simulink model "test12_sudu_pmx_2020a_1"  (R2020a)
settings: Solver=VariableStepAuto  StartTime=0.0  StopTime=100  RelTol=1e-5  AbsTol=1e-5
undefined symbols (not defined in the file or in its folder): Earth, js_decode, js_encode, sigbuilder_block, WGS84
libraries: simulink x14, simulink_extras x7, aerolibfltsims x2, instrumentlib x2, shared6dof x1, aerolibasang x1, aerolibtransform2 x1, aerolibanimutils x1, dspnetwork x1
settings Model: Creator=mx  LastModifiedBy=Platform

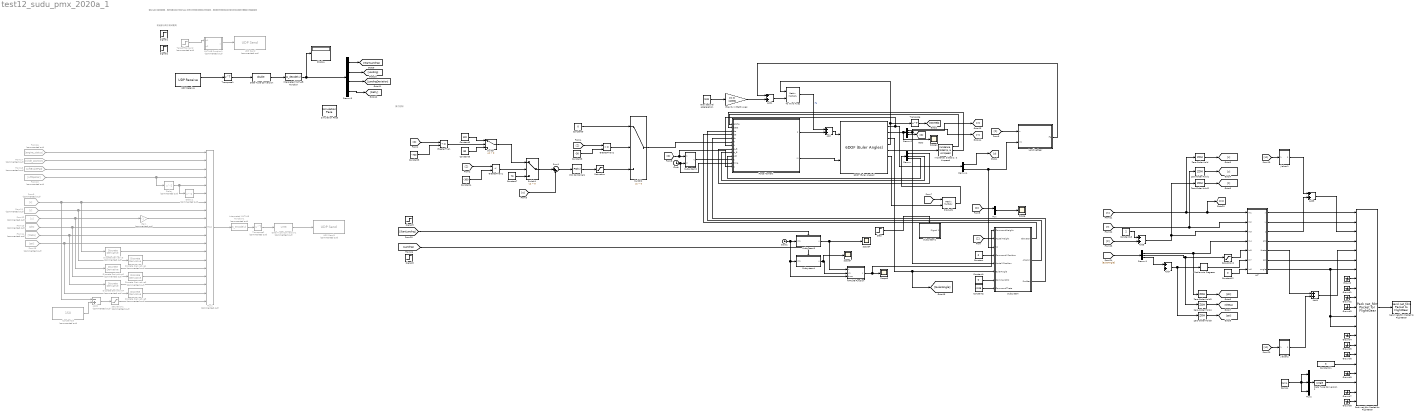
== system test12_sudu_pmx_2020a_1 ==
  note: 推力控制
  note: 通过UDP接收数据，暂时通过自己创造Json的形式来测试是否正常接收，联调的时候将此区域内的发送部分删除只保留接收
  note: 发送部分用于测试使用
  6DOF (Euler Angles) : shared6dof/6DOF (Euler Angles)  units=Metric (MKS)  mtype=Fixed  rep=Euler Angles  xme_0=[0 0 -600]  Vm_0=[80*cosd(-0) 0 80*sind(-0)]  eul_0=[0 -0*pi/180 0]  pm_0=[0 0 0]  mass_0=11000  mass_e=0.5  mass_f=2.0  inertia=[1000,0,0;0,2000,0;0,0,1000]  inertia_e=eye(3)  inertia_f=2*eye(3)  k_quat=1.0  vre_flag=on  abi_flag=off  aMode=0  xme_statename=''  Vm_statename=''  eul_statename=''  quat_statename=''  pm_statename=''  mass_statename=''
      settings: SourceProductBaseCode=AE,PW,MT,UV,VE,VP
  Add{,1,3..5,7} (6 alike) : Sum
  Add2 : Sum  Commented=on  Inputs=-+
  Clock : Clock
  Clock1 : Clock
  Constant{,1,9,12} (4 alike) : Constant  Value=0
  Constant10 : Constant  Commented=on  Value=150
  Constant11 : Constant  Value=3  OutDataTypeStr=uint32
  Constant13 : Constant  Value=2
  Constant2 : Constant  Value=-0.06
  Constant3 : Constant  Value=-700
  Constant4 : Constant  Value=-300
  Constant5 : Constant  Value=80
  Constant6 : Constant  Value=120
  Constant7 : Constant  Value=70
  Constant8 : Constant  Value=-30
  Data Type Conversion : DataTypeConversion  OutDataTypeStr=double
  Data Type Conversion1 : DataTypeConversion  Commented=on  OutDataTypeStr=uint8
  Data Type Conversion2 : DataTypeConversion  OutDataTypeStr=single
  Delay : Delay  Commented=on  InitialCondition=0  SampleTime=1
  Delay1 : Delay  Commented=on  InitialCondition=0  SampleTime=1
  Demux{,1..2,4} (4 alike) : Demux  Outputs=3
  Demux3 : Demux
  Discrete Derivative{,1..5} (6 alike) : simulink/Discrete/Discrete Derivative  Commented=on  gainval=1.0  ICPrevScaledInput=0.0  OutMin=[]  OutMax=[]  OutDataType=fixdt(1, 16)  OutScaling=2^-10  DoSatur=off
  Display : Display
  Force Moment : MATLAB Function  TreatAsAtomicUnit=on
  From10 : From  Commented=on  GotoTag=LiftSpoiler
  From11 : From  Commented=on  GotoTag=y
  From12 : From  Commented=on  GotoTag=z
  From13 : From  Commented=on  GotoTag=phi
  From14 : From  Commented=on  GotoTag=theta
  From15 : From  Commented=on  GotoTag=psi
  From16 : From  Commented=on  GotoTag=engine_status
  From17 : From  Commented=on  GotoTag=slide_position
  From18 : From  Commented=on  GotoTag=LiftBrakePad
  From9 : From  Commented=on  GotoTag=x
  Gain : Gain  Commented=on  Gain=-1
  Gravitational acceleration : Constant  Value=9.81
  Gravity in Earth Axes : Gain  Gain=[0; 0; 11000]  SaturateOnIntegerOverflow=on  OutDataTypeStr=Inherit: Same as input  ParamDataTypeStr=Inherit: Same as input
  GreaterThan : RelationalOperator  Operator=<=  OutDataTypeStr=boolean  RndMeth=Simplest
  GreaterThan1 : RelationalOperator  Operator=<  OutDataTypeStr=boolean  RndMeth=Simplest
  GreaterThan2 : RelationalOperator  OutDataTypeStr=boolean  RndMeth=Simplest
  Ground{,1..9} (10 alike) : Ground
  "Incidence, Sideslip, & Airspeed" : aerolibasang/Incidence, Sideslip, & Airspeed
  Interpreted MATLAB Function : MATLABFcn  MATLABFcn=js_decode(u)
  Interpreted MATLAB Function1 : MATLABFcn  Commented=on  MATLABFcn=js_encode(u)
  LLT : Subsystem
  LandingGear : MATLAB Function  TreatAsAtomicUnit=on
  MATLAB Function : MATLAB Function  TreatAsAtomicUnit=on
  MATLAB Function1 : MATLAB Function  Commented=on  TreatAsAtomicUnit=on
  Mux : Mux  Inputs=2
  Mux1 : Mux  Commented=on  Inputs=19
  Mux2 : Mux  Inputs=3
  PID Controller1 : simulink/Continuous/PID Controller  Controller=PID  Form=Parallel  TimeDomain=Continuous-time  UseExternalTs=off  SampleTime=-1  IntegratorMethod=Forward Euler  FilterMethod=Forward Euler  ControllerParametersSource=internal  P=100000  I=5000  D=10  UseFilter=on  N=10/10  TunerSelectOption=Transfer Function Based (PID Tuner App)  InitialConditionSource=internal  InitialConditionForIntegrator=0  InitialConditionForFilter=0  DifferentiatorICPrevScaledInput=0  ExternalReset=none  TrackingMode=off  Kt=1  LimitOutput=off  UpperSaturationLimit=inf  LowerSaturationLimit=-inf  LinearizeAsGain=on  AntiWindupMode=none  Kb=1  POutMin=[]  POutMax=[]  IOutMin=[]  IOutMax=[]  DOutMin=[]  DOutMax=[]  NOutMin=[]  NOutMax=[]  SumOutMin=[]  SumOutMax=[]  SaturationOutMin=[]  SaturationOutMax=[]  PParamMin=[]  PParamMax=[]  IParamMin=[]  IParamMax=[]  DParamMin=[]  DParamMax=[]  NParamMin=[]  NParamMax=[]  KbParamMin=[]  KbParamMax=[]  KtParamMin=[]  KtParamMax=[]  KbOutMin=[]  KbOutMax=[]  KtOutMin=[]  KtOutMax=[]  IntegratorOutMin=[]  IntegratorOutMax=[]  FilterOutMin=[]  FilterOutMax=[]  SumI1OutMin=[]  SumI1OutMax=[]  SumI2OutMin=[]  SumI2OutMax=[]  SumI3OutMin=[]  SumI3OutMax=[]  SumI4OutMin=[]  SumI4OutMax=[]  SumDOutMin=[]  SumDOutMax=[]  DifferentiatorOutMin=[]  DifferentiatorOutMax=[]  FilterDiffOutCoefMin=[]  FilterDiffOutCoefMax=[]  ReciprocalOutMin=[]  ReciprocalOutMax=[]  SumDenOutMin=[]  SumDenOutMax=[]  SumNumOutMin=[]  SumNumOutMax=[]  DivideOutMin=[]  DivideOutMax=[]  UdiffTsProdOutMin=[]  UdiffTsProdOutMax=[]  NTsProdOutMin=[]  NTsProdOutMax=[]  UintegralTsProdOutMin=[]  UintegralTsProdOutMax=[]  UngainTsProdOutMin=[]  UngainTsProdOutMax=[]  IntegratorContinuousStateAttributes=''  IntegratorStateMustResolveToSignalObject=off  IntegratorRTWStateStorageClass=Auto  FilterContinuousStateAttributes=''  FilterStateMustResolveToSignalObject=off  FilterRTWStateStorageClass=Auto  ParallelPVariant=InternalParameters  IdealPVariant=Disabled  IVariant=InternalParameters  DVariant=InternalParameters  IntegratorVariant=Continuous  SatVariant=Disabled  AWVariant=Passthrough  PCopyVariant=Disabled  TRVariant=Disabled  FdbkBlocksVariant=Forward  IdealPFdbkVariant=Disabled  SatFdbkVariant=Disabled  DerivativeFilterVariant=ContFilter  NVariant=InternalParameters  NCopyVariant=Disabled  FilterICVariant=InternalICsFilter  IntegratorICVariant=InternalICs  ExternalResetVariant=Disabled  TRSumVariant=Passthrough  SumFdbkVariant=Disabled  SumVariant=Sum_PID  TsampFilterVariant=InternalTs  TsampNgainVariant=Passthrough  TsampIntegralVariant=Passthrough
  Pack net_fdm Packet for FlightGear : aerolibfltsims/Pack net_fdm Packet for FlightGear  FlightGearVersion=v2.12  ShowPositionAttitudeInputs=on  ShowVelocityAccelerationInputs=off  ShowControlSurfacePositionInputs=on  ShowEngineFuelInputs=off  ShowLandingGearInputs=on  ShowEnvironmentInputs=off  SampleTime=1/30  packetVersion=24
      settings: SourceProductBaseCode=AE
  Product1 : Product  Multiplication=Matrix(*)
  Radians to Degrees : simulink_extras/Transformations/Radians to Degrees
  Ramp4 : simulink/Sources/Ramp  slope=-0.2  start=20  InitialOutput=1
  Saturation : Saturate  UpperLimit=40000  LowerLimit=0
  Saturation1 : Saturate  Commented=on  UpperLimit=150  LowerLimit=0
  Saturation2 : Saturate  UpperLimit=20
  Scope{,1,3..4,7} (5 alike) : Scope
  Send net_fdm Packet to FlightGear : aerolibfltsims/Send net_fdm Packet to FlightGear  DestinationIpAddress=127.0.0.1  DestinationPort=5502  LocalIpPort=-1  varLen=off  SampleTime=1/30
      settings: SourceProductBaseCode=AE
  Signal1 : Step  Time=2  SampleTime=0
  Signal2 : Step  Time=45  SampleTime=0
  Signal5 : Step  Time=2  SampleTime=0
  Signal8 : Step  Time=45  SampleTime=0
  Simulation Pace : aerolibanimutils/Simulation Pace  SimulationPace=1  SleepMode=Auto  OutputPaceError=off  SampleTime=1
  Step : Step  After=2  SampleTime=0
  Subsystem : Subsystem
  Subsystem1 : Subsystem
  Subsystem2 : Subsystem
  Subsystem3 : Subsystem
  Subsystem4 : Subsystem
  Sum1 : Sum  Inputs=|+-
  Switch : Switch  Criteria=u2 > Threshold
  Switch1 : Switch  Criteria=u2 > Threshold
  Switch2 : Switch  Criteria=u2 > Threshold
  TakeOffComand : Step  Commented=on  Time=6  SampleTime=1
  To Wind Axes : Product  Multiplication=Matrix(*)  InputSameDT=on  SaturateOnIntegerOverflow=on  OutDataTypeStr=Inherit: Same as first input
  Transpose : Math  Operator=transpose  SaturateOnIntegerOverflow=on
  Transpose1 : Math  Operator=transpose  SignedPower=on  SaturateOnIntegerOverflow=on
  Transpose2 : Math  Commented=on  Operator=transpose  SaturateOnIntegerOverflow=on
  UDP Receive : dspnetwork/UDP Receive  localURL='0.0.0.0'  localPort=51001  remoteURL='0.0.0.0'  remotePort=-1  recvBufferSize=8192  dims=992  signalDatatype=uint8  isComplex=off  isVarSize=off  showBlockingTime=off  blockingTime=0  sampletime=1  blockPlatform=[]
  UDP Send : instrumentlib/UDP Send  Commented=on  Host=localhost  Port=51001  LocalPort=-1  EnablePortSharing=off  ByteOrder=BigEndian  OutputDatagramPacketSize=996  EnableBlockingMode=on  LocalAddress=0.0.0.0
  UDP Send1 : instrumentlib/UDP Send  Commented=on  Host=localhost  Port=51003  LocalPort=-1  EnablePortSharing=off  ByteOrder=BigEndian  OutputDatagramPacketSize=1147  EnableBlockingMode=on  LocalAddress=0.0.0.0
  Zero-Order Hold{,1..5} (6 alike) : ZeroOrderHold  SampleTime=-1
  jiaban1 : Subsystem
  jiaban2 : Subsystem
  wires:
  Force Moment/2(M) -> 6DOF (Euler Angles)/2
  6DOF (Euler Angles)/5 -> "Incidence, Sideslip, & Airspeed"/1
  Gravitational acceleration/1 -> Gravity in Earth Axes/1
  To Wind Axes/1 -> Add/1  "Fg"
  Force Moment/1(F) -> Add/2
  Add/1 -> 6DOF (Euler Angles)/1
  "Incidence, Sideslip, & Airspeed"/1 -> Force Moment/1(alpha)
  "Incidence, Sideslip, & Airspeed"/2 -> Force Moment/2(beta)
  6DOF (Euler Angles)/1 -> Demux4/1, Force Moment/7(V)
  Demux/2 -> Force Moment/9(q_B)
  6DOF (Euler Angles)/2 -> Scope1/1, Demux2/1
  6DOF (Euler Angles)/3 -> [EulerAngle], Subsystem/6(EulerAngle)
  Demux4/3 -> LandingGear/2(Vz), Subsystem/3(Vz)
  Mux/1 -> Scope/1
  Constant/1 -> Subsystem/4(CommandYPosition)
  Demux2/2 -> [Y], Subsystem/5(AcutalYPosition)
  Constant1/1 -> Subsystem/7(CommandPsi)
  Constant2/1 -> Subsystem/8(CommandTheta)
  Demux2/3 -> [Z]
  [Z] -> Subsystem/2(AcutalHeight)
  [Z] -> GreaterThan/1
  Constant3/1 -> GreaterThan/2
  Constant4/1 -> GreaterThan1/2
  [Z] -> GreaterThan1/1
  GreaterThan/1 -> Switch/2
  Constant5/1 -> Switch/3
  Constant6/1 -> Switch/1
  GreaterThan1/1 -> Switch1/2
  Constant7/1 -> Switch1/3
  Switch/1 -> Switch1/1
  Switch1/1 -> Sum1/1
  Sum1/1 -> PID Controller1/1
  Demux4/1 -> [u]
  [u] -> Sum1/2
  PID Controller1/1 -> Saturation/1
  Saturation/1 -> Switch2/3
  Constant8/1 -> GreaterThan2/2
  [Z] -> GreaterThan2/1
  GreaterThan2/1 -> Switch2/2
  Constant9/1 -> Switch2/1
  Switch2/1 -> Force Moment/6(T)
  [Z] -> Mux/1
  Subsystem/1(Elevator) -> Force Moment/4(de)
  Subsystem/3(Rudder) -> Force Moment/5(dr)
  Demux/1 -> Force Moment/8(p_B)
  Demux/3 -> Force Moment/10(r_B)
  Subsystem/2(Aileron) -> Force Moment/3(da)
  Transpose/1 -> [DCMeb]
  6DOF (Euler Angles)/4 -> Transpose/1, To Wind Axes/1
  [DCMeb] -> Product1/1
  6DOF (Euler Angles)/6 -> Product1/2
  Product1/1 -> Demux/1
  [Z] -> LandingGear/1(z)
  Gravity in Earth Axes/1 -> Add1/2
  Add1/1 -> To Wind Axes/2
  LandingGear/1(Fe) -> Add1/1
  [Z] -> Force Moment/13(z), Subsystem2/1(z)
  Clock/1 -> Force Moment/12(time), Subsystem2/2(time)
  Subsystem2/1(t) -> Force Moment/11(t)
  Transpose1/1 -> Data Type Conversion/1
  UDP Receive/1 -> Transpose1/1
  MATLAB Function1/1(y) -> UDP Send/1
  Interpreted MATLAB Function/1 -> Demux3/1, Display/1
  TakeOffComand/1 -> MATLAB Function1/1(u1)
  Data Type Conversion/1 -> Interpreted MATLAB Function/1
  Discrete Derivative2/1 -> Mux1/15
  Discrete Derivative1/1 -> Mux1/14
  Delay1/1 -> Mux1/6
  Saturation1/1 -> Mux1/19
  Transpose2/1 -> Data Type Conversion1/1
  Gain/1 -> Mux1/9
  Data Type Conversion1/1 -> UDP Send1/1
  From15/1 -> Discrete Derivative5/1, Mux1/12
  Discrete Derivative/1 -> Mux1/13
  Discrete Derivative5/1 -> Mux1/18
  From16/1 -> Mux1/1
  Delay/1 -> Delay1/1, Mux1/5
  Mux1/1 -> Interpreted MATLAB Function1/1
  From12/1 -> Discrete Derivative2/1, Gain/1
  From9/1 -> Discrete Derivative/1, Mux1/7, Add2/1
  From17/1 -> Mux1/2
  From10/1 -> Delay/1, Mux1/4
  Add2/1 -> Saturation1/1
  From11/1 -> Discrete Derivative1/1, Mux1/8
  Constant10/1 -> Add2/2
  Discrete Derivative4/1 -> Mux1/17
  Discrete Derivative3/1 -> Mux1/16
  Interpreted MATLAB Function1/1 -> Transpose2/1
  From18/1 -> Mux1/3
  From13/1 -> Discrete Derivative3/1, Mux1/10
  From14/1 -> Discrete Derivative4/1, Mux1/11
  Ground/1 -> Pack net_fdm Packet for FlightGear/8
  [x1] -> jiaban2/1(In1)
  LLT/1(x) -> Pack net_fdm Packet for FlightGear/1
  [x1] -> jiaban1/1(In1)
  jiaban1/1(Out1) -> Add3/1
  jiaban2/1(Out1) -> Add4/2
  [Y] -> Zero-Order Hold1/1, LLT/2(In2)
  Zero-Order Hold5/1 -> [psi]
  Radians to Degrees/1 -> LLT/6(In7)
  [X] -> [x1], LLT/1(In1), Zero-Order Hold/1
  Add4/1 -> Pack net_fdm Packet for FlightGear/5
  Add7/1 -> Zero-Order Hold5/1, Radians to Degrees/1
  LLT/7(angle) -> Pack net_fdm Packet for FlightGear/12, Pack net_fdm Packet for FlightGear/13, Pack net_fdm Packet for FlightGear/7
  Data Type Conversion2/1 -> Pack net_fdm Packet for FlightGear/19
  Zero-Order Hold3/1 -> [phi]
  Constant12/1 -> LLT/7(In6)
  Add3/1 -> Pack net_fdm Packet for FlightGear/3
  Zero-Order Hold4/1 -> [theta]
  Ground2/1 -> Pack net_fdm Packet for FlightGear/10
  Zero-Order Hold1/1 -> [y]
  LLT/4(phi) -> Pack net_fdm Packet for FlightGear/4
  Ground8/1 -> Pack net_fdm Packet for FlightGear/21
  Ramp4/1 -> Mux2/3, Mux2/2, Mux2/1
  Ground7/1 -> Pack net_fdm Packet for FlightGear/20
  Constant11/1 -> Pack net_fdm Packet for FlightGear/17
  Zero-Order Hold/1 -> [x]
  Pack net_fdm Packet for FlightGear/1 -> Send net_fdm Packet to FlightGear/1
  Ground6/1 -> Pack net_fdm Packet for FlightGear/16
  Ground3/1 -> Pack net_fdm Packet for FlightGear/11
  Ground4/1 -> Pack net_fdm Packet for FlightGear/14
  Ground5/1 -> Pack net_fdm Packet for FlightGear/15
  Ground1/1 -> Pack net_fdm Packet for FlightGear/9
  Ground9/1 -> Pack net_fdm Packet for FlightGear/18
  LLT/3(z) -> Add3/2
  LLT/2(y) -> Pack net_fdm Packet for FlightGear/2
  LLT/6(psi) -> Pack net_fdm Packet for FlightGear/6
  Zero-Order Hold2/1 -> [z]
  Saturation2/1 -> LLT/5(In5)
  Mux2/1 -> Data Type Conversion2/1
  LLT/5(theta) -> Add4/1
  Demux2/1 -> [X]
  [Z] -> Add5/2
  [EulerAngle] -> Demux1/1
  Demux1/1 -> Zero-Order Hold3/1, LLT/4(In4)
  Demux1/2 -> Zero-Order Hold4/1, Saturation2/1
  Demux1/3 -> Add7/1
  Step/1 -> Subsystem1/Enable
  [StartLanding] -> Subsystem3/Trigger
  Clock1/1 -> Subsystem4/1(In1), MATLAB Function/3(time), Subsystem3/1(In1)
  MATLAB Function/1(y) -> Subsystem/1(CommandHeight), Scope3/1
  Subsystem4/1(u) -> Scope7/1, MATLAB Function/2(u1)
  [Landing] -> Subsystem4/Trigger
  Subsystem3/1(u) -> MATLAB Function/1(u), Scope4/1
  Constant13/1 -> Add5/1
  Add5/1 -> Zero-Order Hold2/1, LLT/3(In3)
  Demux3/1 -> [StartLanding]
  Demux3/2 -> [Landing]
  Demux3/3 -> [LandingDeviation]
  Demux3/4 -> [ReFly]

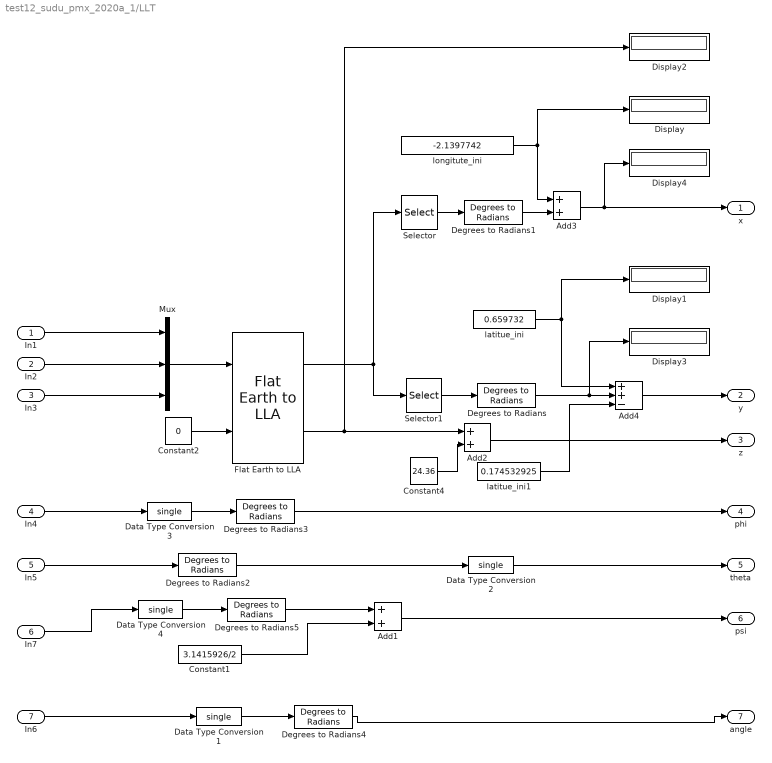
== system test12_sudu_pmx_2020a_1/LLT ==
  In1 : Inport
  In2 : Inport  Port=2
  In3 : Inport  Port=3
  In4 : Inport  Port=4
  In5 : Inport  Port=5
  In7 : Inport  Port=6
  In6 : Inport  Port=7
  Add1 : Sum
  Add2 : Sum
  Add3 : Sum
  Add4 : Sum  Inputs=++-
  Constant1 : Constant  Value=3.1415926/2  OutDataTypeStr=single
  Constant2 : Constant  Value=0
  Constant4 : Constant  Value=24.36
  Data Type Conversion{1..4} (4 alike) : DataTypeConversion  OutDataTypeStr=single
  Degrees to Radians{,1..5} (6 alike) : simulink_extras/Transformations/Degrees to Radians
  Display{,1..4} (5 alike) : Display
  Flat Earth to LLA : aerolibtransform2/Flat Earth to LLA  units=Metric (MKS)  ptype=Earth (WGS84)  F=1/298.257223563  R=6378137  refPosPort=off  LL0=[0 10]  psi=0
  Mux : Mux  Inputs=3
  Selector : Selector  InputPortWidth=2  IndexOptions=Index vector (dialog)  Indices=[1]  OutputSizes=1
  Selector1 : Selector  InputPortWidth=2  IndexOptions=Index vector (dialog)  Indices=[2]  OutputSizes=1
  latitue_ini : Constant  Value=0.659732  OutDataTypeStr=double  LockScale=on
  latitue_ini1 : Constant  Value=0.174532925  OutDataTypeStr=double  LockScale=on
  longitute_ini : Constant  Value=-2.1397742  OutDataTypeStr=double  LockScale=on
  x : Outport
  y : Outport  Port=2
  z : Outport  Port=3
  phi : Outport  Port=4
  theta : Outport  Port=5
  psi : Outport  Port=6
  angle : Outport  Port=7
  wires:
  Degrees to Radians2/1 -> Data Type Conversion2/1
  Degrees to Radians4/1 -> angle/1
  Degrees to Radians1/1 -> Add3/2
  longitute_ini/1 -> Add3/1, Display/1
  In1/1 -> Mux/1
  In2/1 -> Mux/2
  Add3/1 -> x/1, Display4/1
  Flat Earth to LLA/2 -> Add2/1, Display2/1
  Data Type Conversion1/1 -> Degrees to Radians4/1
  latitue_ini/1 -> Add4/1, Display1/1
  Constant4/1 -> Add2/2
  Degrees to Radians/1 -> Add4/2, Display3/1
  latitue_ini1/1 -> Add4/3
  Add4/1 -> y/1
  Add2/1 -> z/1
  Selector1/1 -> Degrees to Radians/1
  Add1/1 -> psi/1
  Flat Earth to LLA/1 -> Selector1/1, Selector/1
  In4/1 -> Data Type Conversion3/1
  Constant1/1 -> Add1/2
  Constant2/1 -> Flat Earth to LLA/2
  In3/1 -> Mux/3
  Selector/1 -> Degrees to Radians1/1
  Mux/1 -> Flat Earth to LLA/1
  In6/1 -> Data Type Conversion1/1
  In5/1 -> Degrees to Radians2/1
  Data Type Conversion2/1 -> theta/1
  Data Type Conversion3/1 -> Degrees to Radians3/1
  Degrees to Radians3/1 -> phi/1
  In7/1 -> Data Type Conversion4/1
  Data Type Conversion4/1 -> Degrees to Radians5/1
  Degrees to Radians5/1 -> Add1/1

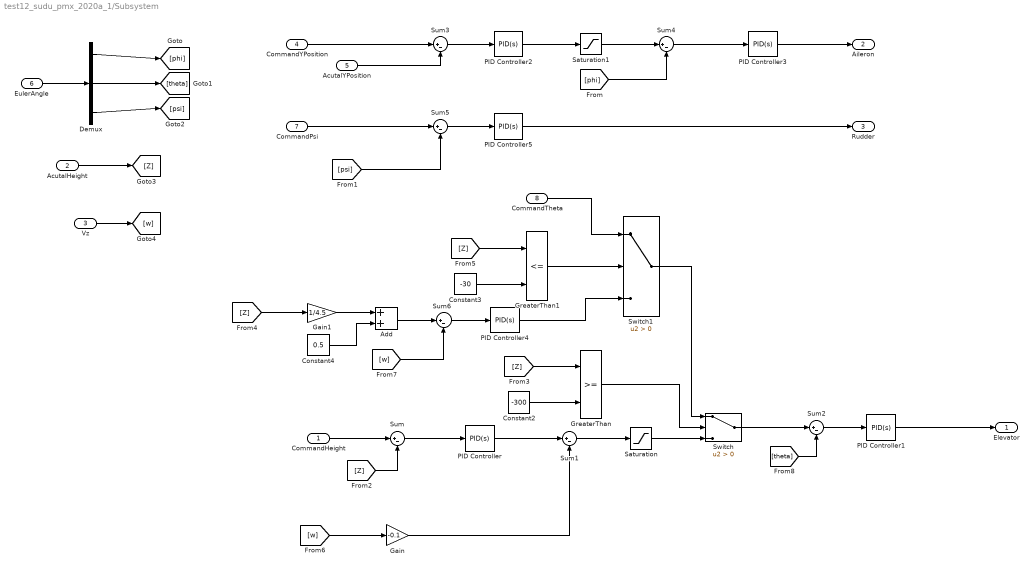
== system test12_sudu_pmx_2020a_1/Subsystem ==
  CommandHeight : Inport
  AcutalHeight : Inport  Port=2
  Vz : Inport  Port=3
  CommandYPosition : Inport  Port=4
  AcutalYPosition : Inport  Port=5
  EulerAngle : Inport  Port=6
  CommandPsi : Inport  Port=7
  CommandTheta : Inport  Port=8
  Add : Sum
  Constant2 : Constant  Value=-300
  Constant3 : Constant  Value=-30
  Constant4 : Constant  Value=0.5
  Demux : Demux  Outputs=3
  Gain : Gain  Gain=-0.1
  Gain1 : Gain  Gain=1/4.5
  GreaterThan : RelationalOperator  OutDataTypeStr=boolean  RndMeth=Simplest
  GreaterThan1 : RelationalOperator  Operator=<=  OutDataTypeStr=boolean  RndMeth=Simplest
  PID Controller : simulink/Continuous/PID Controller  Controller=PID  Form=Parallel  TimeDomain=Continuous-time  UseExternalTs=off  SampleTime=-1  IntegratorMethod=Forward Euler  FilterMethod=Forward Euler  ControllerParametersSource=internal  P=-0.5  I=-0.5/1000  D=-0.5*1000  UseFilter=on  N=1/1000  TunerSelectOption=Transfer Function Based (PID Tuner App)  InitialConditionSource=internal  InitialConditionForIntegrator=0  InitialConditionForFilter=0  DifferentiatorICPrevScaledInput=0  ExternalReset=none  TrackingMode=off  Kt=1  LimitOutput=off  UpperSaturationLimit=inf  LowerSaturationLimit=-inf  LinearizeAsGain=on  AntiWindupMode=none  Kb=1  POutMin=[]  POutMax=[]  IOutMin=[]  IOutMax=[]  DOutMin=[]  DOutMax=[]  NOutMin=[]  NOutMax=[]  SumOutMin=[]  SumOutMax=[]  SaturationOutMin=[]  SaturationOutMax=[]  PParamMin=[]  PParamMax=[]  IParamMin=[]  IParamMax=[]  DParamMin=[]  DParamMax=[]  NParamMin=[]  NParamMax=[]  KbParamMin=[]  KbParamMax=[]  KtParamMin=[]  KtParamMax=[]  KbOutMin=[]  KbOutMax=[]  KtOutMin=[]  KtOutMax=[]  IntegratorOutMin=[]  IntegratorOutMax=[]  FilterOutMin=[]  FilterOutMax=[]  SumI1OutMin=[]  SumI1OutMax=[]  SumI2OutMin=[]  SumI2OutMax=[]  SumI3OutMin=[]  SumI3OutMax=[]  SumI4OutMin=[]  SumI4OutMax=[]  SumDOutMin=[]  SumDOutMax=[]  DifferentiatorOutMin=[]  DifferentiatorOutMax=[]  FilterDiffOutCoefMin=[]  FilterDiffOutCoefMax=[]  ReciprocalOutMin=[]  ReciprocalOutMax=[]  SumDenOutMin=[]  SumDenOutMax=[]  SumNumOutMin=[]  SumNumOutMax=[]  DivideOutMin=[]  DivideOutMax=[]  UdiffTsProdOutMin=[]  UdiffTsProdOutMax=[]  NTsProdOutMin=[]  NTsProdOutMax=[]  UintegralTsProdOutMin=[]  UintegralTsProdOutMax=[]  UngainTsProdOutMin=[]  UngainTsProdOutMax=[]  IntegratorContinuousStateAttributes=''  IntegratorStateMustResolveToSignalObject=off  IntegratorRTWStateStorageClass=Auto  FilterContinuousStateAttributes=''  FilterStateMustResolveToSignalObject=off  FilterRTWStateStorageClass=Auto  ParallelPVariant=InternalParameters  IdealPVariant=Disabled  IVariant=InternalParameters  DVariant=InternalParameters  IntegratorVariant=Continuous  SatVariant=Disabled  AWVariant=Passthrough  PCopyVariant=Disabled  TRVariant=Disabled  FdbkBlocksVariant=Forward  IdealPFdbkVariant=Disabled  SatFdbkVariant=Disabled  DerivativeFilterVariant=ContFilter  NVariant=InternalParameters  NCopyVariant=Disabled  FilterICVariant=InternalICsFilter  IntegratorICVariant=InternalICs  ExternalResetVariant=Disabled  TRSumVariant=Passthrough  SumFdbkVariant=Disabled  SumVariant=Sum_PID  TsampFilterVariant=InternalTs  TsampNgainVariant=Passthrough  TsampIntegralVariant=Passthrough
  PID Controller1 : simulink/Continuous/PID Controller  Controller=PID  Form=Parallel  TimeDomain=Continuous-time  UseExternalTs=off  SampleTime=-1  IntegratorMethod=Forward Euler  FilterMethod=Forward Euler  ControllerParametersSource=internal  P=-100  I=-100/100  D=-100*100  UseFilter=on  N=1/100  TunerSelectOption=Transfer Function Based (PID Tuner App)  InitialConditionSource=internal  InitialConditionForIntegrator=0  InitialConditionForFilter=0  DifferentiatorICPrevScaledInput=0  ExternalReset=none  TrackingMode=off  Kt=1  LimitOutput=off  UpperSaturationLimit=inf  LowerSaturationLimit=-inf  LinearizeAsGain=on  AntiWindupMode=none  Kb=1  POutMin=[]  POutMax=[]  IOutMin=[]  IOutMax=[]  DOutMin=[]  DOutMax=[]  NOutMin=[]  NOutMax=[]  SumOutMin=[]  SumOutMax=[]  SaturationOutMin=[]  SaturationOutMax=[]  PParamMin=[]  PParamMax=[]  IParamMin=[]  IParamMax=[]  DParamMin=[]  DParamMax=[]  NParamMin=[]  NParamMax=[]  KbParamMin=[]  KbParamMax=[]  KtParamMin=[]  KtParamMax=[]  KbOutMin=[]  KbOutMax=[]  KtOutMin=[]  KtOutMax=[]  IntegratorOutMin=[]  IntegratorOutMax=[]  FilterOutMin=[]  FilterOutMax=[]  SumI1OutMin=[]  SumI1OutMax=[]  SumI2OutMin=[]  SumI2OutMax=[]  SumI3OutMin=[]  SumI3OutMax=[]  SumI4OutMin=[]  SumI4OutMax=[]  SumDOutMin=[]  SumDOutMax=[]  DifferentiatorOutMin=[]  DifferentiatorOutMax=[]  FilterDiffOutCoefMin=[]  FilterDiffOutCoefMax=[]  ReciprocalOutMin=[]  ReciprocalOutMax=[]  SumDenOutMin=[]  SumDenOutMax=[]  SumNumOutMin=[]  SumNumOutMax=[]  DivideOutMin=[]  DivideOutMax=[]  UdiffTsProdOutMin=[]  UdiffTsProdOutMax=[]  NTsProdOutMin=[]  NTsProdOutMax=[]  UintegralTsProdOutMin=[]  UintegralTsProdOutMax=[]  UngainTsProdOutMin=[]  UngainTsProdOutMax=[]  IntegratorContinuousStateAttributes=''  IntegratorStateMustResolveToSignalObject=off  IntegratorRTWStateStorageClass=Auto  FilterContinuousStateAttributes=''  FilterStateMustResolveToSignalObject=off  FilterRTWStateStorageClass=Auto  ParallelPVariant=InternalParameters  IdealPVariant=Disabled  IVariant=InternalParameters  DVariant=InternalParameters  IntegratorVariant=Continuous  SatVariant=Disabled  AWVariant=Passthrough  PCopyVariant=Disabled  TRVariant=Disabled  FdbkBlocksVariant=Forward  IdealPFdbkVariant=Disabled  SatFdbkVariant=Disabled  DerivativeFilterVariant=ContFilter  NVariant=InternalParameters  NCopyVariant=Disabled  FilterICVariant=InternalICsFilter  IntegratorICVariant=InternalICs  ExternalResetVariant=Disabled  TRSumVariant=Passthrough  SumFdbkVariant=Disabled  SumVariant=Sum_PID  TsampFilterVariant=InternalTs  TsampNgainVariant=Passthrough  TsampIntegralVariant=Passthrough
  PID Controller2 : simulink/Continuous/PID Controller  Controller=PID  Form=Parallel  TimeDomain=Continuous-time  UseExternalTs=off  SampleTime=-1  IntegratorMethod=Forward Euler  FilterMethod=Forward Euler  ControllerParametersSource=internal  P=0.005  I=0.005/10000  D=0.005*10000  UseFilter=on  N=1/10000  TunerSelectOption=Transfer Function Based (PID Tuner App)  InitialConditionSource=internal  InitialConditionForIntegrator=0  InitialConditionForFilter=0  DifferentiatorICPrevScaledInput=0  ExternalReset=none  TrackingMode=off  Kt=1  LimitOutput=off  UpperSaturationLimit=inf  LowerSaturationLimit=-inf  LinearizeAsGain=on  AntiWindupMode=none  Kb=1  POutMin=[]  POutMax=[]  IOutMin=[]  IOutMax=[]  DOutMin=[]  DOutMax=[]  NOutMin=[]  NOutMax=[]  SumOutMin=[]  SumOutMax=[]  SaturationOutMin=[]  SaturationOutMax=[]  PParamMin=[]  PParamMax=[]  IParamMin=[]  IParamMax=[]  DParamMin=[]  DParamMax=[]  NParamMin=[]  NParamMax=[]  KbParamMin=[]  KbParamMax=[]  KtParamMin=[]  KtParamMax=[]  KbOutMin=[]  KbOutMax=[]  KtOutMin=[]  KtOutMax=[]  IntegratorOutMin=[]  IntegratorOutMax=[]  FilterOutMin=[]  FilterOutMax=[]  SumI1OutMin=[]  SumI1OutMax=[]  SumI2OutMin=[]  SumI2OutMax=[]  SumI3OutMin=[]  SumI3OutMax=[]  SumI4OutMin=[]  SumI4OutMax=[]  SumDOutMin=[]  SumDOutMax=[]  DifferentiatorOutMin=[]  DifferentiatorOutMax=[]  FilterDiffOutCoefMin=[]  FilterDiffOutCoefMax=[]  ReciprocalOutMin=[]  ReciprocalOutMax=[]  SumDenOutMin=[]  SumDenOutMax=[]  SumNumOutMin=[]  SumNumOutMax=[]  DivideOutMin=[]  DivideOutMax=[]  UdiffTsProdOutMin=[]  UdiffTsProdOutMax=[]  NTsProdOutMin=[]  NTsProdOutMax=[]  UintegralTsProdOutMin=[]  UintegralTsProdOutMax=[]  UngainTsProdOutMin=[]  UngainTsProdOutMax=[]  IntegratorContinuousStateAttributes=''  IntegratorStateMustResolveToSignalObject=off  IntegratorRTWStateStorageClass=Auto  FilterContinuousStateAttributes=''  FilterStateMustResolveToSignalObject=off  FilterRTWStateStorageClass=Auto  ParallelPVariant=InternalParameters  IdealPVariant=Disabled  IVariant=InternalParameters  DVariant=InternalParameters  IntegratorVariant=Continuous  SatVariant=Disabled  AWVariant=Passthrough  PCopyVariant=Disabled  TRVariant=Disabled  FdbkBlocksVariant=Forward  IdealPFdbkVariant=Disabled  SatFdbkVariant=Disabled  DerivativeFilterVariant=ContFilter  NVariant=InternalParameters  NCopyVariant=Disabled  FilterICVariant=InternalICsFilter  IntegratorICVariant=InternalICs  ExternalResetVariant=Disabled  TRSumVariant=Passthrough  SumFdbkVariant=Disabled  SumVariant=Sum_PID  TsampFilterVariant=InternalTs  TsampNgainVariant=Passthrough  TsampIntegralVariant=Passthrough
  PID Controller3 : simulink/Continuous/PID Controller  Controller=PID  Form=Parallel  TimeDomain=Continuous-time  UseExternalTs=off  SampleTime=-1  IntegratorMethod=Forward Euler  FilterMethod=Forward Euler  ControllerParametersSource=internal  P=-20  I=-20/100  D=-20*100  UseFilter=on  N=1/100  TunerSelectOption=Transfer Function Based (PID Tuner App)  InitialConditionSource=internal  InitialConditionForIntegrator=0  InitialConditionForFilter=0  DifferentiatorICPrevScaledInput=0  ExternalReset=none  TrackingMode=off  Kt=1  LimitOutput=off  UpperSaturationLimit=inf  LowerSaturationLimit=-inf  LinearizeAsGain=on  AntiWindupMode=none  Kb=1  POutMin=[]  POutMax=[]  IOutMin=[]  IOutMax=[]  DOutMin=[]  DOutMax=[]  NOutMin=[]  NOutMax=[]  SumOutMin=[]  SumOutMax=[]  SaturationOutMin=[]  SaturationOutMax=[]  PParamMin=[]  PParamMax=[]  IParamMin=[]  IParamMax=[]  DParamMin=[]  DParamMax=[]  NParamMin=[]  NParamMax=[]  KbParamMin=[]  KbParamMax=[]  KtParamMin=[]  KtParamMax=[]  KbOutMin=[]  KbOutMax=[]  KtOutMin=[]  KtOutMax=[]  IntegratorOutMin=[]  IntegratorOutMax=[]  FilterOutMin=[]  FilterOutMax=[]  SumI1OutMin=[]  SumI1OutMax=[]  SumI2OutMin=[]  SumI2OutMax=[]  SumI3OutMin=[]  SumI3OutMax=[]  SumI4OutMin=[]  SumI4OutMax=[]  SumDOutMin=[]  SumDOutMax=[]  DifferentiatorOutMin=[]  DifferentiatorOutMax=[]  FilterDiffOutCoefMin=[]  FilterDiffOutCoefMax=[]  ReciprocalOutMin=[]  ReciprocalOutMax=[]  SumDenOutMin=[]  SumDenOutMax=[]  SumNumOutMin=[]  SumNumOutMax=[]  DivideOutMin=[]  DivideOutMax=[]  UdiffTsProdOutMin=[]  UdiffTsProdOutMax=[]  NTsProdOutMin=[]  NTsProdOutMax=[]  UintegralTsProdOutMin=[]  UintegralTsProdOutMax=[]  UngainTsProdOutMin=[]  UngainTsProdOutMax=[]  IntegratorContinuousStateAttributes=''  IntegratorStateMustResolveToSignalObject=off  IntegratorRTWStateStorageClass=Auto  FilterContinuousStateAttributes=''  FilterStateMustResolveToSignalObject=off  FilterRTWStateStorageClass=Auto  ParallelPVariant=InternalParameters  IdealPVariant=Disabled  IVariant=InternalParameters  DVariant=InternalParameters  IntegratorVariant=Continuous  SatVariant=Disabled  AWVariant=Passthrough  PCopyVariant=Disabled  TRVariant=Disabled  FdbkBlocksVariant=Forward  IdealPFdbkVariant=Disabled  SatFdbkVariant=Disabled  DerivativeFilterVariant=ContFilter  NVariant=InternalParameters  NCopyVariant=Disabled  FilterICVariant=InternalICsFilter  IntegratorICVariant=InternalICs  ExternalResetVariant=Disabled  TRSumVariant=Passthrough  SumFdbkVariant=Disabled  SumVariant=Sum_PID  TsampFilterVariant=InternalTs  TsampNgainVariant=Passthrough  TsampIntegralVariant=Passthrough
  PID Controller4 : simulink/Continuous/PID Controller  Controller=PID  Form=Parallel  TimeDomain=Continuous-time  UseExternalTs=off  SampleTime=-1  IntegratorMethod=Forward Euler  FilterMethod=Forward Euler  ControllerParametersSource=internal  P=-0.001  I=-0.001/1000  D=-0.001*100  UseFilter=on  N=1/100  TunerSelectOption=Transfer Function Based (PID Tuner App)  InitialConditionSource=internal  InitialConditionForIntegrator=0  InitialConditionForFilter=0  DifferentiatorICPrevScaledInput=0  ExternalReset=none  TrackingMode=off  Kt=1  LimitOutput=off  UpperSaturationLimit=inf  LowerSaturationLimit=-inf  LinearizeAsGain=on  AntiWindupMode=none  Kb=1  POutMin=[]  POutMax=[]  IOutMin=[]  IOutMax=[]  DOutMin=[]  DOutMax=[]  NOutMin=[]  NOutMax=[]  SumOutMin=[]  SumOutMax=[]  SaturationOutMin=[]  SaturationOutMax=[]  PParamMin=[]  PParamMax=[]  IParamMin=[]  IParamMax=[]  DParamMin=[]  DParamMax=[]  NParamMin=[]  NParamMax=[]  KbParamMin=[]  KbParamMax=[]  KtParamMin=[]  KtParamMax=[]  KbOutMin=[]  KbOutMax=[]  KtOutMin=[]  KtOutMax=[]  IntegratorOutMin=[]  IntegratorOutMax=[]  FilterOutMin=[]  FilterOutMax=[]  SumI1OutMin=[]  SumI1OutMax=[]  SumI2OutMin=[]  SumI2OutMax=[]  SumI3OutMin=[]  SumI3OutMax=[]  SumI4OutMin=[]  SumI4OutMax=[]  SumDOutMin=[]  SumDOutMax=[]  DifferentiatorOutMin=[]  DifferentiatorOutMax=[]  FilterDiffOutCoefMin=[]  FilterDiffOutCoefMax=[]  ReciprocalOutMin=[]  ReciprocalOutMax=[]  SumDenOutMin=[]  SumDenOutMax=[]  SumNumOutMin=[]  SumNumOutMax=[]  DivideOutMin=[]  DivideOutMax=[]  UdiffTsProdOutMin=[]  UdiffTsProdOutMax=[]  NTsProdOutMin=[]  NTsProdOutMax=[]  UintegralTsProdOutMin=[]  UintegralTsProdOutMax=[]  UngainTsProdOutMin=[]  UngainTsProdOutMax=[]  IntegratorContinuousStateAttributes=''  IntegratorStateMustResolveToSignalObject=off  IntegratorRTWStateStorageClass=Auto  FilterContinuousStateAttributes=''  FilterStateMustResolveToSignalObject=off  FilterRTWStateStorageClass=Auto  ParallelPVariant=InternalParameters  IdealPVariant=Disabled  IVariant=InternalParameters  DVariant=InternalParameters  IntegratorVariant=Continuous  SatVariant=Disabled  AWVariant=Passthrough  PCopyVariant=Disabled  TRVariant=Disabled  FdbkBlocksVariant=Forward  IdealPFdbkVariant=Disabled  SatFdbkVariant=Disabled  DerivativeFilterVariant=ContFilter  NVariant=InternalParameters  NCopyVariant=Disabled  FilterICVariant=InternalICsFilter  IntegratorICVariant=InternalICs  ExternalResetVariant=Disabled  TRSumVariant=Passthrough  SumFdbkVariant=Disabled  SumVariant=Sum_PID  TsampFilterVariant=InternalTs  TsampNgainVariant=Passthrough  TsampIntegralVariant=Passthrough
  PID Controller5 : simulink/Continuous/PID Controller  Controller=PID  Form=Parallel  TimeDomain=Continuous-time  UseExternalTs=off  SampleTime=-1  IntegratorMethod=Forward Euler  FilterMethod=Forward Euler  ControllerParametersSource=internal  P=-0.5  I=-0.5/1  D=-0.5*1  UseFilter=on  N=1/1  TunerSelectOption=Transfer Function Based (PID Tuner App)  InitialConditionSource=internal  InitialConditionForIntegrator=0  InitialConditionForFilter=0  DifferentiatorICPrevScaledInput=0  ExternalReset=none  TrackingMode=off  Kt=1  LimitOutput=off  UpperSaturationLimit=inf  LowerSaturationLimit=-inf  LinearizeAsGain=on  AntiWindupMode=none  Kb=1  POutMin=[]  POutMax=[]  IOutMin=[]  IOutMax=[]  DOutMin=[]  DOutMax=[]  NOutMin=[]  NOutMax=[]  SumOutMin=[]  SumOutMax=[]  SaturationOutMin=[]  SaturationOutMax=[]  PParamMin=[]  PParamMax=[]  IParamMin=[]  IParamMax=[]  DParamMin=[]  DParamMax=[]  NParamMin=[]  NParamMax=[]  KbParamMin=[]  KbParamMax=[]  KtParamMin=[]  KtParamMax=[]  KbOutMin=[]  KbOutMax=[]  KtOutMin=[]  KtOutMax=[]  IntegratorOutMin=[]  IntegratorOutMax=[]  FilterOutMin=[]  FilterOutMax=[]  SumI1OutMin=[]  SumI1OutMax=[]  SumI2OutMin=[]  SumI2OutMax=[]  SumI3OutMin=[]  SumI3OutMax=[]  SumI4OutMin=[]  SumI4OutMax=[]  SumDOutMin=[]  SumDOutMax=[]  DifferentiatorOutMin=[]  DifferentiatorOutMax=[]  FilterDiffOutCoefMin=[]  FilterDiffOutCoefMax=[]  ReciprocalOutMin=[]  ReciprocalOutMax=[]  SumDenOutMin=[]  SumDenOutMax=[]  SumNumOutMin=[]  SumNumOutMax=[]  DivideOutMin=[]  DivideOutMax=[]  UdiffTsProdOutMin=[]  UdiffTsProdOutMax=[]  NTsProdOutMin=[]  NTsProdOutMax=[]  UintegralTsProdOutMin=[]  UintegralTsProdOutMax=[]  UngainTsProdOutMin=[]  UngainTsProdOutMax=[]  IntegratorContinuousStateAttributes=''  IntegratorStateMustResolveToSignalObject=off  IntegratorRTWStateStorageClass=Auto  FilterContinuousStateAttributes=''  FilterStateMustResolveToSignalObject=off  FilterRTWStateStorageClass=Auto  ParallelPVariant=InternalParameters  IdealPVariant=Disabled  IVariant=InternalParameters  DVariant=InternalParameters  IntegratorVariant=Continuous  SatVariant=Disabled  AWVariant=Passthrough  PCopyVariant=Disabled  TRVariant=Disabled  FdbkBlocksVariant=Forward  IdealPFdbkVariant=Disabled  SatFdbkVariant=Disabled  DerivativeFilterVariant=ContFilter  NVariant=InternalParameters  NCopyVariant=Disabled  FilterICVariant=InternalICsFilter  IntegratorICVariant=InternalICs  ExternalResetVariant=Disabled  TRSumVariant=Passthrough  SumFdbkVariant=Disabled  SumVariant=Sum_PID  TsampFilterVariant=InternalTs  TsampNgainVariant=Passthrough  TsampIntegralVariant=Passthrough
  Saturation : Saturate  UpperLimit=0.3  LowerLimit=-0.3
  Saturation1 : Saturate  UpperLimit=0.3  LowerLimit=-0.3
  Sum{,1..6} (7 alike) : Sum  Inputs=|+-
  Switch : Switch  Criteria=u2 > Threshold
  Switch1 : Switch  Criteria=u2 > Threshold
  Elevator : Outport
  Aileron : Outport  Port=2
  Rudder : Outport  Port=3
  wires:
  Sum/1 -> PID Controller/1
  Gain/1 -> Sum1/2
  Sum1/1 -> Saturation/1
  PID Controller/1 -> Sum1/1
  PID Controller1/1 -> Elevator/1
  Sum2/1 -> PID Controller1/1
  [theta] -> Sum2/2
  [w] -> Gain/1
  CommandHeight/1 -> Sum/1
  CommandYPosition/1 -> Sum3/1
  AcutalYPosition/1 -> Sum3/2
  Sum3/1 -> PID Controller2/1
  PID Controller2/1 -> Saturation1/1
  Saturation1/1 -> Sum4/1
  EulerAngle/1 -> Demux/1
  Demux/1 -> [phi]
  Demux/2 -> [theta]
  Demux/3 -> [psi]
  [phi] -> Sum4/2
  Sum4/1 -> PID Controller3/1
  PID Controller3/1 -> Aileron/1
  CommandPsi/1 -> Sum5/1
  [psi] -> Sum5/2
  Sum5/1 -> PID Controller5/1
  PID Controller5/1 -> Rudder/1
  Saturation/1 -> Switch/3
  AcutalHeight/1 -> [Z]
  [Z] -> Sum/2
  [Z] -> GreaterThan/1
  Constant2/1 -> GreaterThan/2
  GreaterThan/1 -> Switch/2
  Switch1/1 -> Switch/1
  Constant3/1 -> GreaterThan1/2
  [Z] -> GreaterThan1/1
  GreaterThan1/1 -> Switch1/2
  [Z] -> Gain1/1
  Gain1/1 -> Add/1
  Constant4/1 -> Add/2
  Add/1 -> Sum6/1
  Vz/1 -> [w]
  [w] -> Sum6/2
  Sum6/1 -> PID Controller4/1
  PID Controller4/1 -> Switch1/3
  CommandTheta/1 -> Switch1/1
  Switch/1 -> Sum2/1

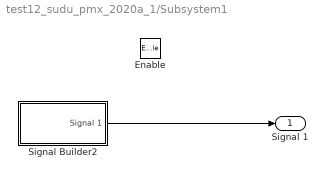
== system test12_sudu_pmx_2020a_1/Subsystem1 ==
  Enable : EnablePort
  Signal Builder2 : Subsystem  Tag=STV Subsys  LoadFcn=sigbuilder_block('load');  StartFcn=sigbuilder_block('start');  StopFcn=sigbuilder_block('stop');  ClipboardFcn=sigbuilder_block('clipboard');  mask(Sigbuilder block){tuvar=[0:10]}
      mask help: Simulink:masks:SigbuilderBlock_MD
      mask init:
      | if ~strcmp(get_param(bdroot(gcbh),'SimulationStatus'),'stopped') tuvar = sigbuilder_block('maskInit'); end
      settings: CopyFcn=sigbuilder_block('copy');  DeleteFcn=sigbuilder_block('delete');  ModelCloseFcn=sigbuilder_block('modelClose');  PreSaveFcn=sigbuilder_block('preSave');  PauseFcn=sigbuilder_block('pause');  ContinueFcn=sigbuilder_block('continue');  NameChangeFcn=sigbuilder_block('namechange');  OpenFcn=sigbuilder_block('open',[12 45 1006.5 318.75 ]);  CloseFcn=sigbuilder_block('close');
      mask Display: plot(0, 0, 100, 100,[2, 2, 32, 32, 2], [68, 8, 8, 68, 68],[32, 2], [38, 38], [32, 19, 2],[53, 60, 44], [32, 17, 17, 2],[16, 16, 31, 31]);txt = getActiveGroup(gcbh);text(2, 100, txt,'verticalAlignment', 'top');
  Signal 1 : Outport  InitialOutput=-600
  wires:
  Signal Builder2/1(Signal 1) -> Signal 1/1

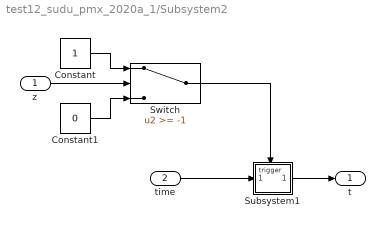
== system test12_sudu_pmx_2020a_1/Subsystem2 ==
  z : Inport
  time : Inport  Port=2
  Constant : Constant
  Constant1 : Constant  Value=0
  Subsystem1 : Subsystem
  Switch : Switch  Threshold=-1
  t : Outport
  wires:
  time/1 -> Subsystem1/1(In1)
  Subsystem1/1(Out1) -> t/1
  z/1 -> Switch/2
  Constant/1 -> Switch/1
  Constant1/1 -> Switch/3
  Switch/1 -> Subsystem1/Trigger

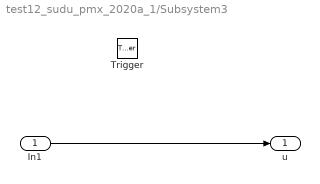
== system test12_sudu_pmx_2020a_1/Subsystem3 ==
  In1 : Inport
  Trigger : TriggerPort  VariantControl=Variant  PortDimensions=1
  u : Outport
  wires:
  In1/1 -> u/1

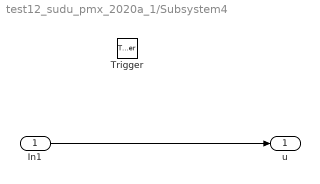
== system test12_sudu_pmx_2020a_1/Subsystem4 ==
  In1 : Inport
  Trigger : TriggerPort  VariantControl=Variant  PortDimensions=1
  u : Outport
  wires:
  In1/1 -> u/1

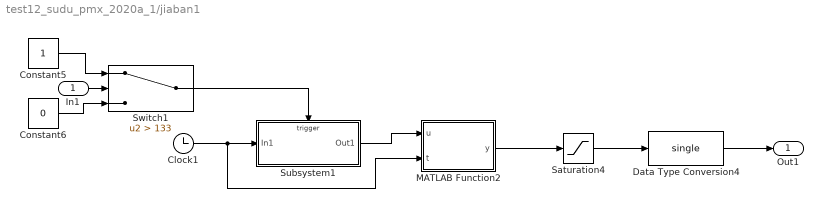
== system test12_sudu_pmx_2020a_1/jiaban1 ==
  In1 : Inport
  Clock1 : Clock
  Constant5 : Constant
  Constant6 : Constant  Value=0
  Data Type Conversion4 : DataTypeConversion  OutDataTypeStr=single
  MATLAB Function2 : MATLAB Function  TreatAsAtomicUnit=on
  Saturation4 : Saturate  UpperLimit=20
  Subsystem1 : Subsystem
  Switch1 : Switch  Criteria=u2 > Threshold  Threshold=133
  Out1 : Outport
  wires:
  MATLAB Function2/1(y) -> Saturation4/1
  Clock1/1 -> MATLAB Function2/2(t), Subsystem1/1(In1)
  Constant5/1 -> Switch1/1
  Switch1/1 -> Subsystem1/Trigger
  In1/1 -> Switch1/2
  Saturation4/1 -> Data Type Conversion4/1
  Subsystem1/1(Out1) -> MATLAB Function2/1(u)
  Constant6/1 -> Switch1/3
  Data Type Conversion4/1 -> Out1/1

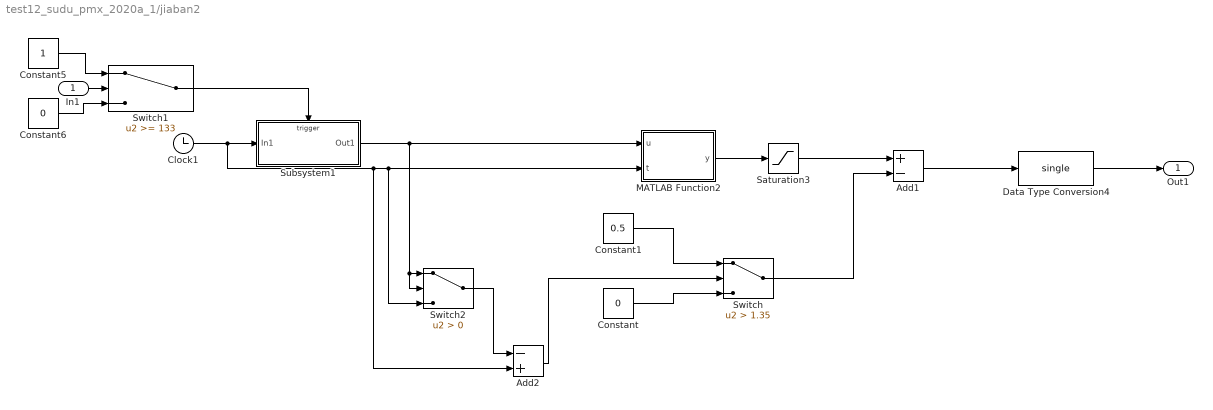
== system test12_sudu_pmx_2020a_1/jiaban2 ==
  In1 : Inport
  Add1 : Sum  Inputs=+-
  Add2 : Sum  Inputs=-+
  Clock1 : Clock
  Constant : Constant  Value=0
  Constant1 : Constant  Value=0.5
  Constant5 : Constant
  Constant6 : Constant  Value=0
  Data Type Conversion4 : DataTypeConversion  OutDataTypeStr=single
  MATLAB Function2 : MATLAB Function  TreatAsAtomicUnit=on
  Saturation3 : Saturate
  Subsystem1 : Subsystem
  Switch : Switch  Criteria=u2 > Threshold  Threshold=1.35
  Switch1 : Switch  Threshold=133
  Switch2 : Switch  Criteria=u2 > Threshold
  Out1 : Outport
  wires:
  Constant6/1 -> Switch1/3
  Subsystem1/1(Out1) -> Switch2/1, Switch2/2, MATLAB Function2/1(u)
  In1/1 -> Switch1/2
  Switch1/1 -> Subsystem1/Trigger
  Constant5/1 -> Switch1/1
  Clock1/1 -> Subsystem1/1(In1), Add2/2, Switch2/3, MATLAB Function2/2(t)
  MATLAB Function2/1(y) -> Saturation3/1
  Constant/1 -> Switch/3
  Constant1/1 -> Switch/1
  Switch/1 -> Add1/2
  Saturation3/1 -> Add1/1
  Add1/1 -> Data Type Conversion4/1
  Data Type Conversion4/1 -> Out1/1
  Switch2/1 -> Add2/1
  Add2/1 -> Switch/2

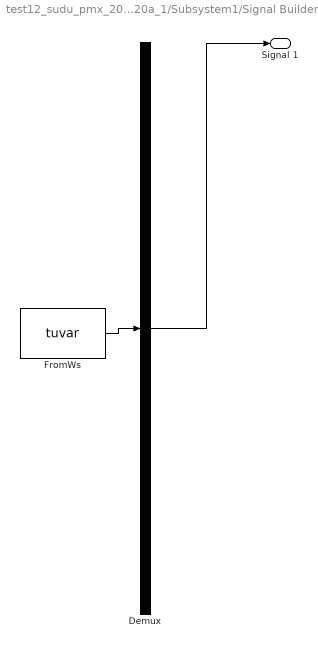
== system test12_sudu_pmx_2020a_1/Subsystem1/Signal Builder2 ==
  Demux : Demux  Tag=STV Demux  Outputs=1
      settings: DisplayOption=none
  FromWs : FromWorkspace  Tag=STV FromWs  VariableName=tuvar
      SigBuilderData=|
      | common.afterFinalStr = 'Extrapolate'
      | common.sampleTime = 0
      | dataSet.timeRange = [0 100]
      | dataSet.name = 'Group 1'
      | sbobj.Groups.Name = 'Group 1'
      | sbobj.Groups.Signals.Name = 'Signal 1'
      | sbobj.Groups.Signals.XData = [0 2 3 50 64 100]
      | sbobj.Groups.Signals.YData = [-600 -600 -600 -290 0 0]
      | sbobj.Groups.TimeRange = [0 100]
  Signal 1 : Outport  Tag=STV Outport
  wires:
  Demux/1 -> Signal 1/1
  FromWs/1 -> Demux/1

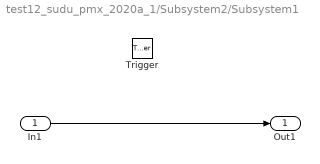
== system test12_sudu_pmx_2020a_1/Subsystem2/Subsystem1 ==
  In1 : Inport
  Trigger : TriggerPort  VariantControl=Variant  PortDimensions=1
  Out1 : Outport  InitialOutput=100
  wires:
  In1/1 -> Out1/1

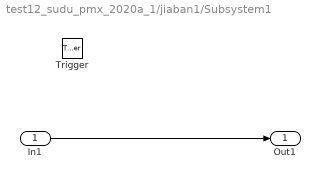
== system test12_sudu_pmx_2020a_1/jiaban1/Subsystem1 ==
  In1 : Inport
  Trigger : TriggerPort  VariantControl=Variant  PortDimensions=1
  Out1 : Outport
  wires:
  In1/1 -> Out1/1

== system test12_sudu_pmx_2020a_1/jiaban2/Subsystem1 ==
  In1 : Inport
  Trigger : TriggerPort  VariantControl=Variant  PortDimensions=1
  Out1 : Outport
  wires:
  In1/1 -> Out1/1

== matlab function test12_sudu_pmx_2020a_1/LandingGear ==
  data: z input; Fe output; Vz input
function Fe = fcn(z,Vz)
h = -z;
Vh = -Vz;
c = 300000*4;
d = 100000*4;
contact = h < 0;
if contact
    fc = -c*abs(h);
    fd2 = d*Vh;
else
    fc = 0;
    fd2 = 0;
end
if contact
    if fd2 < fc 
        fd = fc;
    elseif fd2 > -fc
        fd = -fc;
    else
        fd = fd2;
    end
else
    fd = 0;
end
Fe = zeros(3,1);
Fe(1) = 0;
Fe(2) = 0;
Fe(3) = fc + fd;

== matlab function test12_sudu_pmx_2020a_1/Force Moment ==
  data: alpha input; beta input; da input; de input; dr input; T input; F output; V input; p_B input; M output; q_B input; r_B input; t input; time input; z input
function [F,M] = fcn(alpha,beta,da,de,dr,T,V,p_B,q_B,r_B,t,time,z)
cbar=10;
lt=10;
St=5;
S=20;
rho=1.22505;
V_A = norm(V);
q_dyn=rho/2.0*V_A*V_A;
qS=q_dyn*S;
cLwb_alpha=3.5;
alpha0=5*pi/180;
cLwb=cLwb_alpha*(alpha + alpha0);
cLt_alpha=1.5;
epps=0.25*(alpha + alpha0);
alpha_tail=alpha - epps+ de + 1.3*q_B*lt/V_A;
cLt=cLt_alpha*alpha_tail*St/S;
cL=cLwb+cLt;
cD_0=0.03;
cD_cL_min=0.15;
cD_cL2=0.07;
cD=cD_0+cD_cL2*(cLwb-cD_cL_min)^2;
cY_beta=-1.6;
cY_rudder=0.24;
cY=cY_beta*beta+cY_rudder*dr;
Tbs=[cos(alpha)*cos(beta),-cos(alpha)*sin(beta),-sin(alpha);...
     sin(beta),            cos(beta),          0;...
     sin(alpha)*cos(beta),-sin(alpha)*sin(beta),cos(alpha)];
F_S=qS.*[-cD;cY;-cL];
F_B=Tbs*F_S+[T;0;0];
if time >= t 
    if V(1) >= 1e-8 && z >=-1 
        F_brake = -11000*27; 
    else
        F_brake = 0;
    end
else
    F_brake = 0;
end
F = zeros(3,1);  
if z <= -100
    F(1)=F_B(1) - 11000*2
else
    F(1)=F_B(1) + F_brake;
end
F(2)=F_B(2);
F(3)=F_B(3);
cl_beta=-1.4;
cm_0=-0.59;
cn_beta=1;
cn_alphabeta=-1/15.0*180/pi;
clmn0=[cl_beta*beta;    cm_0 - cLt*lt/cbar;     cn_beta*beta + cn_alphabeta*alpha*beta];
clmnRot=[-11.0,     0,    5.0;...
         0,    -5,      0;...
         1.7,     0,  -11.5];
clmnAct=[ -0.6,     0,   0.22;...
         0,   -10,      0;...
         0,     0,  -0.63];
clmn=clmn0+clmnRot*[p_B;q_B;r_B]*cbar/V_A+clmnAct*[da;de;dr];
M_B=qS*cbar*clmn;
M = zeros(3,1);
M(1)=M_B(1);
M(2)=M_B(2);
M(3)=M_B(3);

end

== matlab function test12_sudu_pmx_2020a_1/MATLAB Function1 ==
  data: y output uint8; u1 input; u2 input
function  y = json_encode(u1,u2)
S = struct("StartLanding",...
            struct("id", 1,"type","int","data", u1,"dirction","IN","info","ToMatlab,0_NotAllowed,1_Allowed"),...
            "Landing",....
            struct("id", 2,"type","int","data", u2,"dirction","IN","info","ToMatlab,0_null,1_start"),...
            "LandingDeviation",....
            struct("id", 3,"type","data","data", [1,2,3],"dirction","IN","info","ToMatlab,Landing Deviation Information"),...
            "ReFly",....
            struct("id", 4,"type","int","data", 0,"dirction","IN","info","ToMatlab,ReFly Information"));
coder.extrinsic('jsonencode');
result = jsonencode(S);
y = uint8(zeros(1,992));
y =  uint8(result);

== matlab function test12_sudu_pmx_2020a_1/MATLAB Function ==
  data: u input; u1 input; y output; time input
function y = fcn(u,u1,time)
if u <= 0 
    y = -600;
else
    if time < (u+2)
        y = -600;
    elseif time <= (u+2+47)
        if u1 > 0 
            if time < u1 + 2       
                y = (time-u-2)*(-290+600)/(50-3)-600;
            else
                y_ini = (u1+2-u-2)*(-290+600)/(50-3)-600;
                y = (time-u1-2)*290/(64-50) + y_ini;            
            end
        else
           y = (time-u-2)*(-290+600)/(50-3)-600; 
        end
    elseif time <= (u+2+47+14)
        if u1 > 0
            y_ini = (u1+2-u-2)*(-290+600)/(50-3)-600;
            y = (time-u1-2)*290/(64-50) + y_ini;
        else
            y = (time-u-2-47)*290/(64-50)-290;
        end
    else
        y = 0;
    end
    if y >= 0
        y = 0;
    end
end

== matlab function test12_sudu_pmx_2020a_1/jiaban1/MATLAB Function2 ==
  data: u input; y output; t input
function y = fcn(u,t)
if u <= 0
    start_time = 0;
    y = 0;
else
    start_time = u;
    y = (t-start_time)*15;
end

== matlab function test12_sudu_pmx_2020a_1/jiaban2/MATLAB Function2 ==
  data: u input; y output; t input
function y = fcn(u,t)
if u <= 0
    start_time = 0;
    y = 0;
else
    start_time = u;
    y = (t-start_time)*4;
end
